simulink model "dom1"  (R2017b)
settings: Solver=ode45  StartTime=0.0  StopTime=50  MaxStep=0.01  RelTol=1e-5  EnableMultiTasking=on
settings Model: Creator=John Whittington  LastModifiedBy=niquit
settings DataIOCC: LimitDataPoints=on  SaveFormat=Array  SignalLoggingSaveFormat=ModelDataLogs
settings OptimizationCC: ExpressionDepthLimit=2147483647  LifeSpan=inf
settings DebuggingCC: UnderspecifiedInitializationDetection=Classic  MergeDetectMultiDrivingBlocksExec=none  SolverPrmCheckMsg=warning  FcnCallInpInsideContextMsg=warning  StateNameClashWarn=warning  SFUnexpectedBacktrackingDiag=warning  SFNoUnconditionalDefaultTransitionDiag=warning  SFExecutionAtInitializationDiag=none
settings HardwareCC: ProdBitPerPointer=32  ProdBitPerSizeT=32  ProdBitPerPtrDiffT=32  ProdLargestAtomicFloat=None  ProdIntDivRoundTo=Undefined  ProdEndianess=Unspecified  ProdWordSize=32  ProdHWDeviceType=32-bit Generic
settings ModelReferenceCC: PropagateSignalLabelsOutOfModel=off
settings CodeAppCC: StateflowObjectComments=on
settings GRTTargetCC: TargetLangStandard=C89/C90 (ANSI)  GeneratePreprocessorConditionals=Disable all  CombineOutputUpdateFcns=off  GRTInterface=on
settings ConfigComp: CovMetricSettings=dw  CovHtmlReporting=on  CovSaveCumulativeToWorkspaceVar=on  CovSaveSingleToWorkspaceVar=on  CovExternalEMLEnable=off

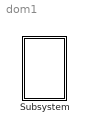
== system dom1 ==
  Subsystem : Subsystem  mask{M1=1, M2=2, L1=1, L2=2, fi1=180, fi2=50, g=9.81, T=0}

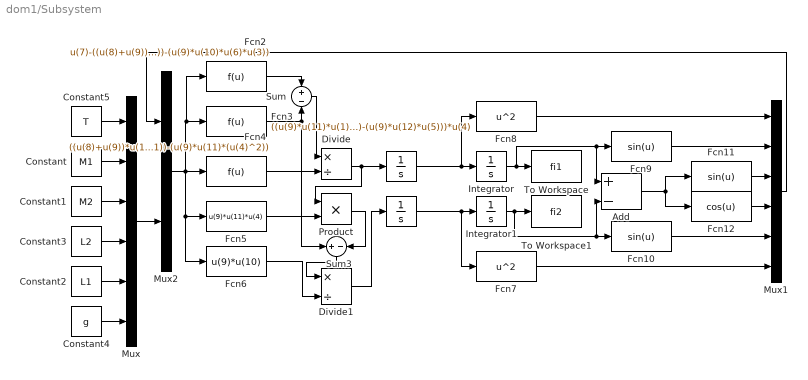
== system dom1/Subsystem ==
  " " : Integrator
  " " : Integrator
  Add : Sum  Inputs=+-
  Constant : Constant  Value=M1
  Constant1 : Constant  Value=M2
  Constant2 : Constant  Value=L1
  Constant3 : Constant  Value=L2
  Constant4 : Constant  Value=g
  Constant5 : Constant  Value=T
  Divide : Product  Inputs=*/
  Divide1 : Product  Inputs=*/
  Fcn10 : Fcn  Expr=sin(u)
  Fcn11 : Fcn  Expr=sin(u)
  Fcn12 : Fcn  Expr=cos(u)
  Fcn2 : Fcn  Expr=u(7)-((u(8)+u(9))*u(12)*u(2))-(u(9)*u(10)*u(6)*u(3))
  Fcn3 : Fcn  Expr=((u(9)*u(11)*u(1)*u(3))-(u(9)*u(12)*u(5)))*u(4)
  Fcn4 : Fcn  Expr=((u(8)+u(9))*u(11))-(u(9)*u(11)*(u(4)^2))
  Fcn5 : Fcn  Expr=u(9)*u(11)*u(4)
  Fcn6 : Fcn  Expr=u(9)*u(10)
  Fcn7 : Fcn  Expr=u^2
  Fcn8 : Fcn  Expr=u^2
  Fcn9 : Fcn  Expr=sin(u)
  Integrator : Integrator  InitialCondition=fi1*pi/180
  Integrator1 : Integrator  InitialCondition=fi2*pi/180
  Mux : Mux  Inputs=6
  Mux1 : Mux  Inputs=6
  Mux2 : Mux  Inputs=2
  Product : Product  RndMeth=Zero
  Sum : Sum  Inputs=+-
  Sum3 : Sum  Inputs=+-
  To Workspace : ToWorkspace  VariableName=fi1  SampleTime=-1
      settings: Save2DSignal=2-D array (concatenate along first dimension)
  To Workspace1 : ToWorkspace  VariableName=fi2  SampleTime=-1
      settings: Save2DSignal=2-D array (concatenate along first dimension)
  wires:
  " "/1 -> Integrator1/1, Fcn7/1
  Product/1 -> Sum3/2
  Constant2/1 -> Mux/5
  Mux/1 -> Mux2/2
  Mux2/1 -> Fcn3/1, Fcn2/1, Fcn6/1, Fcn5/1, Fcn4/1
  Divide1/1 -> " "/1
  Fcn2/1 -> Sum/1
  Mux1/1 -> Mux2/1
  Fcn7/1 -> Mux1/6
  Constant4/1 -> Mux/6
  Fcn10/1 -> Mux1/5
  Constant3/1 -> Mux/4
  Constant5/1 -> Mux/1
  Add/1 -> Fcn12/1, Fcn11/1
  Fcn3/1 -> Sum3/1, Sum/2
  Fcn8/1 -> Mux1/1
  " "/1 -> Integrator/1, Fcn8/1
  Sum/1 -> Divide/1
  Fcn5/1 -> Product/2
  Integrator1/1 -> To Workspace1/1, Add/2, Fcn10/1
  Integrator/1 -> Fcn9/1, Add/1, To Workspace/1
  Constant1/1 -> Mux/3
  Fcn6/1 -> Divide1/2
  Fcn12/1 -> Mux1/4
  Fcn11/1 -> Mux1/3
  Fcn4/1 -> Divide/2
  Fcn9/1 -> Mux1/2
  Sum3/1 -> Divide1/1
  Constant/1 -> Mux/2
  Divide/1 -> Product/1, " "/1
